simulink model "a3_anti_roll_control_sim"  (R2022b)
settings: Solver=VariableStepAuto  StartTime=0.0  StopTime=20  RelTol=1e-3
values from neighbouring files (symbols this model uses):
  qhalf = halfLinearModel(ms,mus_fl,mus_fr,k_fl,k_fr,c_fl,c_fr,kt_fl,kt_fr,kb,t_f,Ix,actuator)    [a3_half_car_control.m]
undefined symbols (not defined in the file or in its folder): hinfK
settings Model: Creator=phatdo  LastModifiedBy=phatdo
settings DataIOCC: ReturnWorkspaceOutputs=off

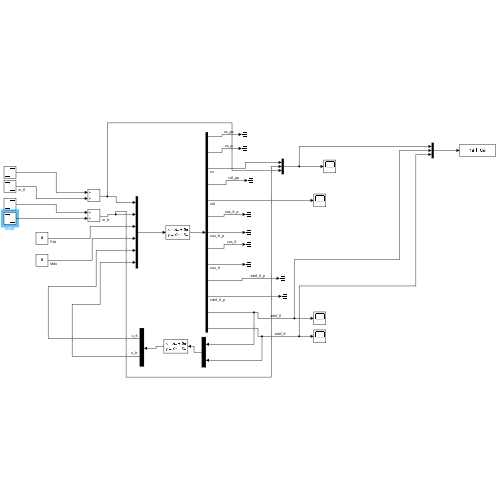
[thumbnail: Simulink's stored preview of the top-level diagram]
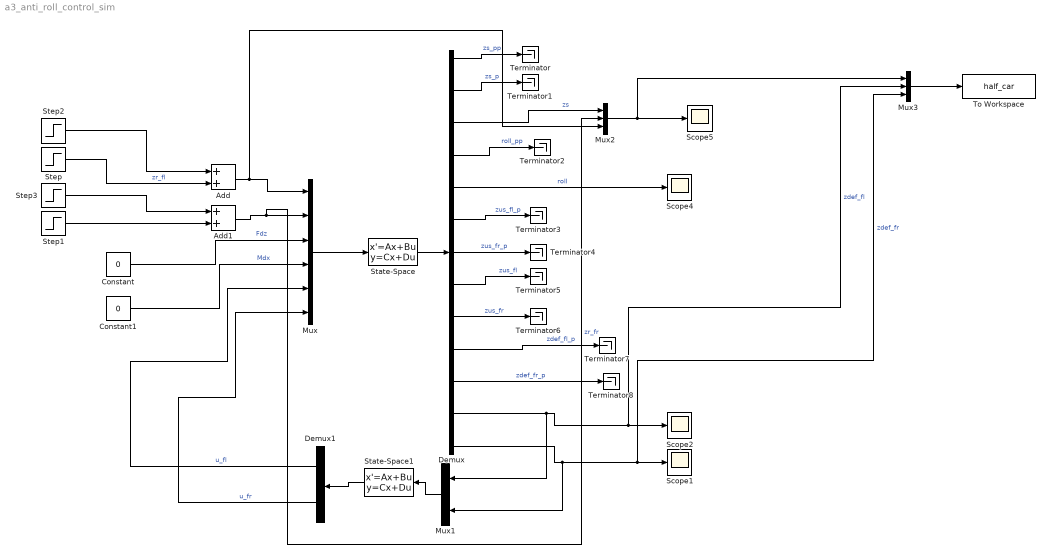
== system a3_anti_roll_control_sim ==
  Add : Sum
  Add1 : Sum
  Constant : Constant  Value=0
  Constant1 : Constant  Value=0
  Demux : Demux  Outputs=13
  Demux1 : Demux  Outputs=2
  Mux : Mux  Inputs=6
  Mux1 : Mux  Inputs=2
  Mux2 : Mux  Inputs=3
  Mux3 : Mux  Inputs=3
  Scope{1..2,4..5} (4 alike) : Scope
  State-Space : StateSpace  A=qhalf.a  B=qhalf.b  C=qhalf.c  D=qhalf.d  InitialCondition=0
  State-Space1 : StateSpace  A=hinfK.a  B=hinfK.b  C=hinfK.c  D=hinfK.d  InitialCondition=0
  Step : Step  Time=3  After=-.01  SampleTime=0
  Step1 : Step  Time=8  After=-.01  SampleTime=0
  Step2 : Step  After=.01  SampleTime=0
  Step3 : Step  Time=5  After=.01  SampleTime=0
  Terminator{,1..8} (9 alike) : Terminator
  To Workspace : ToWorkspace  VariableName=half_car  SaveFormat=Timeseries  SampleTime=-1
  wires:
  Demux/8 -> Terminator5/1  "zus_fl"
  Demux/3 -> Mux2/1  "zs"
  Mux/1 -> State-Space/1
  Demux/11 -> Terminator8/1  "zdef_fr_p"
  Constant/1 -> Mux/3  "Fdz"
  Step3/1 -> Add1/1
  State-Space1/1 -> Demux1/1
  Add/1 -> Mux2/3, Mux/1
  Demux/5 -> Scope4/1  "roll"
  Add1/1 -> Mux2/2, Mux/2  "zr_fr"
  Mux1/1 -> State-Space1/1
  Demux/13 -> Scope1/1, Mux3/3, Mux1/2  "zdef_fr"
  Demux1/1 -> Mux/5  "u_fl"
  Demux/10 -> Terminator7/1  "zdef_fl_p"
  Step1/1 -> Add1/2
  Demux/12 -> Mux3/2, Scope2/1, Mux1/1  "zdef_fl"
  Step2/1 -> Add/1
  State-Space/1 -> Demux/1
  Demux/7 -> Terminator4/1  "zus_fr_p"
  Demux/4 -> Terminator2/1  "roll_pp"
  Step/1 -> Add/2  "zr_fl"
  Constant1/1 -> Mux/4  "Mdx"
  Demux/1 -> Terminator/1  "zs_pp"
  Demux/6 -> Terminator3/1  "zus_fl_p"
  Mux3/1 -> To Workspace/1
  Demux/2 -> Terminator1/1  "zs_p"
  Mux2/1 -> Mux3/1, Scope5/1
  Demux1/2 -> Mux/6  "u_fr"
  Demux/9 -> Terminator6/1  "zus_fr"
